simulink model "CONTROLLO_ADATTATIVO"  (R2020b)
settings: Solver=ode1  StartTime=0.0  StopTime=T(end)+3  FixedStep=0.001  RelTol=1e-3
undefined symbols (not defined in the file): a1, a2, d0, DiscIntNeverNeededParam, KD_ad, LAMBDA, param_esatti, pi0, q0
settings Model: Creator=pc  LastModifiedBy=Utente

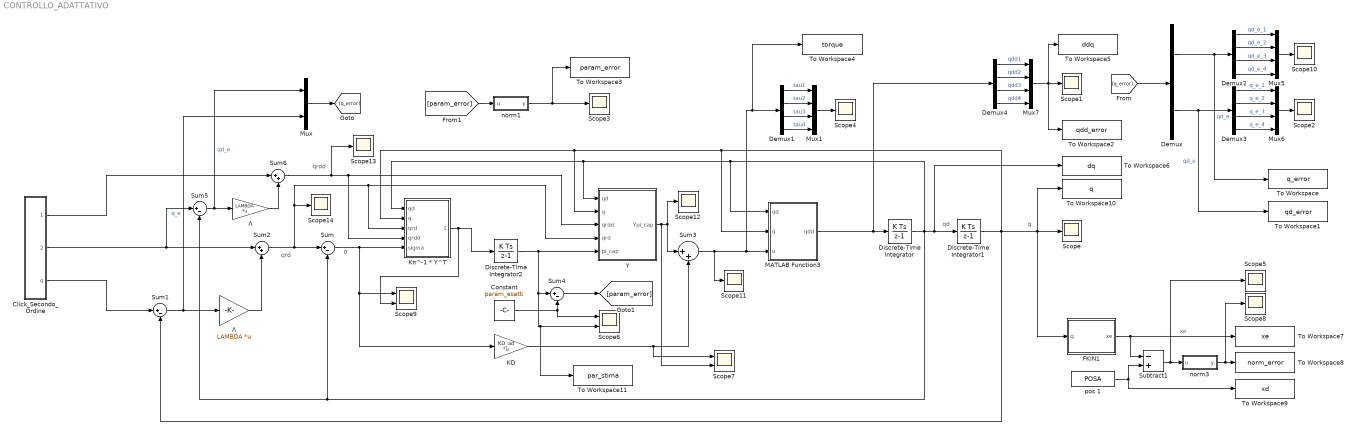
== system CONTROLLO_ADATTATIVO ==
  note: qd
  note: qrd
  note: qrdd
  note: q
  note: σ
  Click_Secondo_Ordine : Subsystem
  Constant : Constant  Value=param_esatti
  Demux : Demux  Outputs=2
  Demux{1..4} (4 alike) : Demux
  Discrete-Time Integrator : DiscreteIntegrator  InitialCondition=[0 0 0 0]  SampleTime=0.001  ICPrevOutput=DiscIntNeverNeededParam  ICPrevScaledInput=DiscIntNeverNeededParam
  Discrete-Time Integrator1 : DiscreteIntegrator  InitialCondition=q0  SampleTime=0.001  ICPrevOutput=DiscIntNeverNeededParam  ICPrevScaledInput=DiscIntNeverNeededParam
  Discrete-Time Integrator2 : DiscreteIntegrator  gainval=1  InitialCondition=pi0  SampleTime=0.001  ICPrevOutput=DiscIntNeverNeededParam  ICPrevScaledInput=DiscIntNeverNeededParam
  FKIN1 : MATLAB Function  TreatAsAtomicUnit=on
  KD : Gain  Gain=KD_ad  Multiplication=Matrix(K*u) (u vector)
  Kπ^-1 * Y^T : MATLAB Function  TreatAsAtomicUnit=on
  MATLAB Function3 : MATLAB Function  TreatAsAtomicUnit=on
  Mux : Mux  Inputs=2
  Mux{1,5..7} (4 alike) : Mux
  Scope{,1..5,8,10..14} (12 alike) : Scope
  Scope6 : Scope  NumInputPorts=2
  Scope7 : Scope  NumInputPorts=2
  Scope9 : Scope  NumInputPorts=2
  Subtract1 : Sum  Inputs=-+
  Sum{,1,4..5} (4 alike) : Sum  Inputs=|+-
  Sum2 : Sum  Inputs=|++
  Sum3 : Sum  Inputs=|++
  Sum6 : Sum  Inputs=|++
  To Workspace : ToWorkspace  VariableName=q_error  SaveFormat=Timeseries  SampleTime=-1
  To Workspace1 : ToWorkspace  VariableName=qd_error  SaveFormat=Timeseries  SampleTime=-1
  To Workspace10 : ToWorkspace  VariableName=q  SaveFormat=Timeseries  SampleTime=-1
  To Workspace11 : ToWorkspace  VariableName=par_stima  SaveFormat=Timeseries  SampleTime=-1
  To Workspace2 : ToWorkspace  VariableName=qdd_error  SaveFormat=Timeseries  SampleTime=-1
  To Workspace3 : ToWorkspace  VariableName=param_error  SaveFormat=Timeseries  SampleTime=-1
  To Workspace4 : ToWorkspace  VariableName=torque  SaveFormat=Timeseries  SampleTime=-1
  To Workspace5 : ToWorkspace  VariableName=ddq  SaveFormat=Timeseries  SampleTime=-1
  To Workspace6 : ToWorkspace  VariableName=dq  SaveFormat=Timeseries  SampleTime=-1
  To Workspace7 : ToWorkspace  VariableName=xe  SaveFormat=Timeseries  SampleTime=-1
  To Workspace8 : ToWorkspace  VariableName=norm_error  SaveFormat=Timeseries  SampleTime=-1
  To Workspace9 : ToWorkspace  VariableName=xd  SaveFormat=Timeseries  SampleTime=-1
  Y : MATLAB Function  TreatAsAtomicUnit=on
  norm1 : MATLAB Function  TreatAsAtomicUnit=on
  norm3 : MATLAB Function  TreatAsAtomicUnit=on
  pos 1 : FromWorkspace  VariableName=POSA  SampleTime=0.001  OutputAfterFinalValue=Holding final value
  Λ : Gain  Gain=LAMBDA  Multiplication=Matrix(K*u) (u vector)
  "Λ " : Gain  Gain=LAMBDA  Multiplication=Matrix(K*u) (u vector)
  wires:
  Sum6/1 -> Scope13/1, Y/3(qrdd), Kπ^-1 * Y^T/4(qrdd)
  Discrete-Time Integrator2/1 -> To Workspace11/1, Scope6/2, Sum4/1, Y/5(pi_cap)
  "Λ "/1 -> Sum6/2
  Kπ^-1 * Y^T/1(pi_capd) -> Scope9/2, Discrete-Time Integrator2/1
  Sum3/1 -> Scope11/1, To Workspace4/1, Demux1/1, MATLAB Function3/3(u)
  Y/1(Ypi_cap) -> Scope7/2, Sum3/1, Scope12/1
  Click_Secondo_Ordine/3(q) -> Sum1/1
  Sum/1 -> Scope9/1, KD/1, Kπ^-1 * Y^T/5(sigma)
  Click_Secondo_Ordine/2(q_d) -> Sum5/1, Sum2/1
  KD/1 -> Scope7/1, Sum3/2
  Λ/1 -> Sum2/2
  Click_Secondo_Ordine/1(q_dd) -> Sum6/1
  Sum2/1 -> Scope14/1, Y/4(qrd), Kπ^-1 * Y^T/3(qrd), Sum/1
  Demux4/1 -> Mux7/1  "qdd1"
  Demux4/2 -> Mux7/2  "qdd2"
  Demux4/3 -> Mux7/3  "qdd3"
  Demux1/3 -> Mux1/3  "tau3"
  Demux1/4 -> Mux1/4  "tau4"
  Mux1/1 -> Scope4/1
  Mux7/1 -> To Workspace5/1, To Workspace2/1, Scope1/1
  Discrete-Time Integrator/1 -> To Workspace6/1, Discrete-Time Integrator1/1, Y/1(qd), Kπ^-1 * Y^T/1(qd), MATLAB Function3/1(qd), Sum5/2, Sum/2
  Demux1/2 -> Mux1/2  "tau2"
  Demux4/4 -> Mux7/4  "qdd4"
  Demux1/1 -> Mux1/1  "tau1"
  MATLAB Function3/1(qdd) -> Demux4/1, Discrete-Time Integrator/1
  Mux/1 -> [q_error]
  Sum1/1 -> Mux/2, Λ/1  "q_e"
  Sum5/1 -> Mux/1, "Λ "/1  "qd_e"
  Mux6/1 -> Scope2/1
  Mux5/1 -> Scope10/1
  Demux3/3 -> Mux6/3  "q_e_3"
  Demux3/4 -> Mux6/4  "q_e_4"
  [q_error] -> Demux/1
  Demux3/1 -> Mux6/1  "q_e_1"
  Demux3/2 -> Mux6/2  "q_e_2"
  Demux2/3 -> Mux5/3  "qd_e_3"
  Demux2/4 -> Mux5/4  "qd_e_4"
  Demux/1 -> To Workspace/1, Demux2/1  "qd_e"
  Demux2/2 -> Mux5/2  "qd_e_2"
  Demux/2 -> To Workspace1/1, Demux3/1  "qd_e"
  Demux2/1 -> Mux5/1  "qd_e_1"
  Discrete-Time Integrator1/1 -> Y/2(q), Kπ^-1 * Y^T/2(q), MATLAB Function3/2(q), To Workspace10/1, FKIN1/1(q), Scope/1, Sum1/2
  [param_error] -> norm1/1(u)
  norm3/1(y) -> Scope8/1, To Workspace8/1
  pos 1/1 -> Subtract1/2, To Workspace9/1
  FKIN1/1(xe) -> Subtract1/1, To Workspace7/1  "xe"
  Subtract1/1 -> Scope5/1, norm3/1(u)
  Constant/1 -> Scope6/1, Sum4/2
  Sum4/1 -> [param_error]
  norm1/1(y) -> To Workspace3/1, Scope3/1

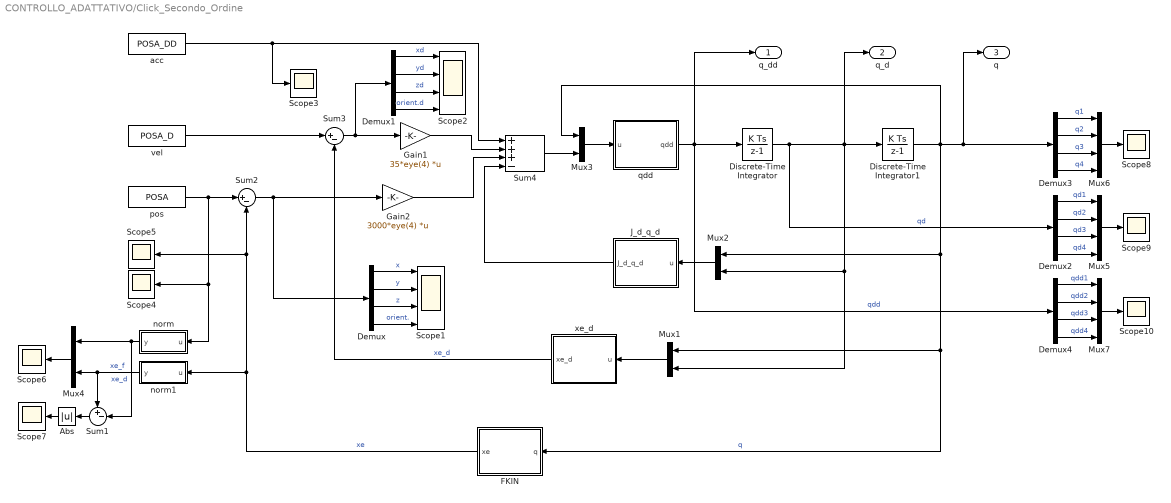
== system CONTROLLO_ADATTATIVO/Click_Secondo_Ordine ==
  Abs : Abs
  Demux{,1..4} (5 alike) : Demux
  Discrete-Time Integrator : DiscreteIntegrator  InitialCondition=zeros(1,4)  SampleTime=1e-3  ICPrevOutput=DiscIntNeverNeededParam  ICPrevScaledInput=DiscIntNeverNeededParam
  Discrete-Time Integrator1 : DiscreteIntegrator  InitialCondition=q0  SampleTime=1e-3  ICPrevOutput=DiscIntNeverNeededParam  ICPrevScaledInput=DiscIntNeverNeededParam
  FKIN : MATLAB Function  TreatAsAtomicUnit=on
  Gain1 : Gain  Gain=35*eye(4)  Multiplication=Matrix(K*u)
  Gain2 : Gain  Gain=3000*eye(4)  Multiplication=Matrix(K*u)
  J_d_q_d : MATLAB Function  TreatAsAtomicUnit=on
  Mux{1..4} (4 alike) : Mux  Inputs=2
  Mux5 : Mux
  Mux6 : Mux
  Mux7 : Mux
  Scope1 : Scope  NumInputPorts=4
  Scope{3..10} (8 alike) : Scope
  Scope2 : Scope  NumInputPorts=4
  Sum1 : Sum  Inputs=+-|
  Sum2 : Sum  Inputs=|+-
  Sum3 : Sum  Inputs=|+-
  Sum4 : Sum  Inputs=+++-
  acc : FromWorkspace  VariableName=POSA_DD  SampleTime=0.001
  norm : MATLAB Function  TreatAsAtomicUnit=on
  norm1 : MATLAB Function  TreatAsAtomicUnit=on
  "pos " : FromWorkspace  VariableName=POSA  SampleTime=0.001
  qdd : MATLAB Function  TreatAsAtomicUnit=on
  "vel " : FromWorkspace  VariableName=POSA_D  SampleTime=0.001
  xe_d : MATLAB Function  TreatAsAtomicUnit=on
  q_dd : Outport
  q_d : Outport  Port=2
  q : Outport  Port=3
  wires:
  Mux1/1 -> xe_d/1(u)
  J_d_q_d/1(J_d_q_d) -> Sum4/4
  "vel "/1 -> Sum3/1
  "pos "/1 -> norm/1(u), Scope4/1, Sum2/1
  Sum2/1 -> Demux/1, Gain2/1
  Sum3/1 -> Demux1/1, Gain1/1
  Discrete-Time Integrator1/1 -> Demux3/1, q/1, Mux3/1, Mux2/1, Mux1/1, FKIN/1(q)  "q"
  Mux2/1 -> J_d_q_d/1(u)
  xe_d/1(xe_d) -> Sum3/2  "xe_d"
  Mux3/1 -> qdd/1(u)
  Gain2/1 -> Sum4/3
  qdd/1(qdd) -> Demux4/1, q_dd/1, Discrete-Time Integrator/1  "qdd"
  FKIN/1(xe) -> Sum2/2, Scope5/1, norm1/1(u)  "xe"
  Discrete-Time Integrator/1 -> Demux2/1, q_d/1, Mux2/2, Mux1/2, Discrete-Time Integrator1/1  "qd"
  Sum4/1 -> Mux3/2
  acc/1 -> Sum4/1, Scope3/1
  Gain1/1 -> Sum4/2
  Abs/1 -> Scope7/1
  norm1/1(y) -> Sum1/1, Mux4/2  "xe_f"
  norm/1(y) -> Sum1/2, Mux4/1  "xe_d"
  Sum1/1 -> Abs/1
  Mux4/1 -> Scope6/1
  Demux/4 -> Scope1/4  "orient."
  Demux/2 -> Scope1/2  "y"
  Demux/1 -> Scope1/1  "x"
  Demux/3 -> Scope1/3  "z"
  Demux1/4 -> Scope2/4  "orient.d"
  Demux1/2 -> Scope2/2  "yd"
  Demux1/1 -> Scope2/1  "xd"
  Demux1/3 -> Scope2/3  "zd"
  Demux2/3 -> Mux5/3  "qd3"
  Demux3/1 -> Mux6/1  "q1"
  Mux5/1 -> Scope9/1
  Demux3/2 -> Mux6/2  "q2"
  Demux2/2 -> Mux5/2  "qd2"
  Demux3/4 -> Mux6/4  "q4"
  Demux2/1 -> Mux5/1  "qd1"
  Mux6/1 -> Scope8/1
  Demux3/3 -> Mux6/3  "q3"
  Demux2/4 -> Mux5/4  "qd4"
  Demux4/4 -> Mux7/4  "qdd4"
  Demux4/2 -> Mux7/2  "qdd2"
  Demux4/1 -> Mux7/1  "qdd1"
  Mux7/1 -> Scope10/1
  Demux4/3 -> Mux7/3  "qdd3"

== matlab function CONTROLLO_ADATTATIVO/Click_Secondo_Ordine/norm ==
  data: u input; y output
function y = norm(u)
y = norm(u);

== matlab function CONTROLLO_ADATTATIVO/Click_Secondo_Ordine/norm1 ==
  data: u input; y output
function y = norm(u)
y = norm(u);

== matlab function CONTROLLO_ADATTATIVO/norm3 ==
  data: u input; y output
function y = fcn(u)
y = norm(u);

== matlab function CONTROLLO_ADATTATIVO/Y ==
  data: qd input; q input; qrdd input; qrd input; pi_cap input; Ypi_cap output
function Ypi_cap = fcn(qd, q, qrdd, qrd, pi_cap)

q_1 = q(1);
q_2 = q(2);
q_3 = q(3);
q_4 = q(4);
qd_1 = qd(1);
qd_2 = qd(2);
qd_3 = qd(3);
qd_4 = qd(4);
q_rdd_1=qrdd(1);
q_rdd_2=qrdd(2);
q_rdd_3=qrdd(3);
q_rdd_4=qrdd(4);
q_rd_1=qrd(1);
q_rd_2=qrd(2);
q_rd_3=qrd(3);
q_rd_4=qrd(4);

Y=[q_rdd_1/16, q_rdd_1, q_rdd_1, q_rd_1, q_rdd_1*(cos(q_2)/4 + 5/16) + q_rdd_2*(cos(q_2)/8 + 1/16) - (q_rd_1*qd_2*sin(q_2))/8 - (q_rd_2*sin(q_2)*(qd_1 + qd_2))/8, q_rdd_1 + q_rdd_2, q_rdd_1 + q_rdd_2,      0, q_rdd_1*(cos(q_2)/2 + 1/2) + q_rdd_2*(cos(q_2)/4 + 1/4) - (q_rd_1*qd_2*sin(q_2))/4 - (q_rd_2*sin(q_2)*(qd_1 + qd_2))/4, q_rdd_1 + q_rdd_2,         q_rdd_1 + q_rdd_2 + 50*q_rdd_3,          0, q_rdd_1*(cos(q_2)/2 + 1/2) + q_rdd_2*(cos(q_2)/4 + 1/4) - (q_rd_1*qd_2*sin(q_2))/4 - (q_rd_2*sin(q_2)*(qd_1 + qd_2))/4, q_rdd_1 + q_rdd_2 + q_rdd_4,        q_rdd_1 + q_rdd_2 + 20*q_rdd_4,          0;
     0,       0,       0,      0,                                                      q_rdd_2/16 + q_rdd_1*(cos(q_2)/8 + 1/16) + (q_rd_1*qd_1*sin(q_2))/8, q_rdd_1 + q_rdd_2, q_rdd_1 + q_rdd_2, q_rd_2,                                                      q_rdd_2/4 + q_rdd_1*(cos(q_2)/4 + 1/4) + (q_rd_1*qd_1*sin(q_2))/4, q_rdd_1 + q_rdd_2,         q_rdd_1 + q_rdd_2 + 50*q_rdd_3,          0,                                                      q_rdd_2/4 + q_rdd_1*(cos(q_2)/4 + 1/4) + (q_rd_1*qd_1*sin(q_2))/4, q_rdd_1 + q_rdd_2 + q_rdd_4,        q_rdd_1 + q_rdd_2 + 20*q_rdd_4,          0;
     0,       0,       0,      0,                                                                                                                        0,                 0,                 0,      0,                                                                                                      q_rdd_3 + 981/100,                 0, 50*q_rdd_1 + 50*q_rdd_2 + 2500*q_rdd_3, 400*q_rd_3,                                                                                                      q_rdd_3 + 981/100,                           0,                                     0,          0;
        0,       0,       0,      0,                                                                                                                        0,                 0,                 0,      0,                                                                                                                      0,                 0,                                      0,          0,                                                                                                                      0, q_rdd_1 + q_rdd_2 + q_rdd_4, 20*q_rdd_1 + 20*q_rdd_2 + 400*q_rdd_4, 400*q_rd_4];

    
Ypi_cap = Y*pi_cap;

== matlab function CONTROLLO_ADATTATIVO/Kπ^-1 * Y^T ==
  data: qd input; q input; qrd input; qrdd input; sigma input; pi_capd output; Kpi parameter
function pi_capd = fcn(qd, q, qrd, qrdd, sigma, Kpi)

q_1 = q(1);
q_2 = q(2);
q_3 = q(3);
q_4 = q(4);
qd_1 = qd(1);
qd_2 = qd(2);
qd_3 = qd(3);
qd_4 = qd(4);
q_rd_1 = qrd(1);
q_rd_2 = qrd(2);
q_rd_3 = qrd(3);
q_rd_4 = qrd(4);
q_rdd_1 = qrdd(1);
q_rdd_2 = qrdd(2);
q_rdd_3 = qrdd(3);
q_rdd_4 = qrdd(4);

Y=[q_rdd_1/16, q_rdd_1, q_rdd_1, q_rd_1, q_rdd_1*(cos(q_2)/4 + 5/16) + q_rdd_2*(cos(q_2)/8 + 1/16) - (q_rd_1*qd_2*sin(q_2))/8 - (q_rd_2*sin(q_2)*(qd_1 + qd_2))/8, q_rdd_1 + q_rdd_2, q_rdd_1 + q_rdd_2,      0, q_rdd_1*(cos(q_2)/2 + 1/2) + q_rdd_2*(cos(q_2)/4 + 1/4) - (q_rd_1*qd_2*sin(q_2))/4 - (q_rd_2*sin(q_2)*(qd_1 + qd_2))/4, q_rdd_1 + q_rdd_2,         q_rdd_1 + q_rdd_2 + 50*q_rdd_3,          0, q_rdd_1*(cos(q_2)/2 + 1/2) + q_rdd_2*(cos(q_2)/4 + 1/4) - (q_rd_1*qd_2*sin(q_2))/4 - (q_rd_2*sin(q_2)*(qd_1 + qd_2))/4, q_rdd_1 + q_rdd_2 + q_rdd_4,        q_rdd_1 + q_rdd_2 + 20*q_rdd_4,          0;
     0,       0,       0,      0,                                                      q_rdd_2/16 + q_rdd_1*(cos(q_2)/8 + 1/16) + (q_rd_1*qd_1*sin(q_2))/8, q_rdd_1 + q_rdd_2, q_rdd_1 + q_rdd_2, q_rd_2,                                                      q_rdd_2/4 + q_rdd_1*(cos(q_2)/4 + 1/4) + (q_rd_1*qd_1*sin(q_2))/4, q_rdd_1 + q_rdd_2,         q_rdd_1 + q_rdd_2 + 50*q_rdd_3,          0,                                                      q_rdd_2/4 + q_rdd_1*(cos(q_2)/4 + 1/4) + (q_rd_1*qd_1*sin(q_2))/4, q_rdd_1 + q_rdd_2 + q_rdd_4,        q_rdd_1 + q_rdd_2 + 20*q_rdd_4,          0;
     0,       0,       0,      0,                                                                                                                        0,                 0,                 0,      0,                                                                                                      q_rdd_3 + 981/100,                 0, 50*q_rdd_1 + 50*q_rdd_2 + 2500*q_rdd_3, 400*q_rd_3,                                                                                                      q_rdd_3 + 981/100,                           0,                                     0,          0;
        0,       0,       0,      0,                                                                                                                        0,                 0,                 0,      0,                                                                                                                      0,                 0,                                      0,          0,                                                                                                                      0, q_rdd_1 + q_rdd_2 + q_rdd_4, 20*q_rdd_1 + 20*q_rdd_2 + 400*q_rdd_4, 400*q_rd_4];

    
pi_capd = inv(Kpi)* Y' * sigma;

== matlab function CONTROLLO_ADATTATIVO/FKIN1 ==
  data: q input; xe output; a2 parameter; a1 parameter; d0 parameter
function xe = fcn(q, a2, a1, d0)

theta1 = q(1);
theta2 = q(2);
d3 = q(3);
theta4 = q(4);

% Cinematica diretta
xe = [a1*cos(theta1)+a2*cos(theta1+theta2) ;
      a1*sin(theta1)+a2*sin(theta1+theta2) ;
      d3+d0;
      theta1+theta2+theta4; ];
end

== matlab function CONTROLLO_ADATTATIVO/MATLAB Function3 ==
  data: qd input; q input; u input; qdd output
function qdd = manipulator(qd, q, u)

q_1 = q(1);
q_2 = q(2);
q_3 = q(3);
q_4 = q(4);
qd_1 = qd(1);
qd_2 = qd(2);
qd_3 = qd(3);
qd_4 = qd(4);

l1 = 0.25;
l2 = 0.25;
ml1 = 25;   %Massa dal giunto 1 al giunto 2 .Non si considera quello della base.
ml2 = ml1;
ml3 = 10;
ml4 = 5; 


Il1 = 5;
Il2 = Il1;
Il3 = 0;
Il4 = 1;


mm = zeros(1,4);

%Costanti di trasmissione meccanica 
kr1 = 1;
kr2 = kr1;
kr3 = 50;
kr4 = 20;


Im1 = 0.02;
Im2 = Im1;
Im3 = 0.005;
Im4 = 0.001;


Fm1= 0.0001;
Fm2 = Fm1;
Fm3 = 0.01;
Fm4 = 0.005;

   
n = [ Fm1*qd_1 - (qd_2*sin(q_2)*(qd_1 + qd_2)*(ml2 + 2*ml3 + 2*ml4))/8 - qd_1*qd_2*sin(q_2)*(ml2/8 + ml3/4 + ml4/4);
                                                 sin(q_2)*(ml2/8 + ml3/4 + ml4/4)*qd_1^2 + Fm2*qd_2;
                                                                  (981*ml3)/100 + (981*ml4)/100 + 400*Fm3*qd_3;
                                                                             400*Fm4*qd_4];
 
                                                                    
B = [ Il1 + Il2 + Il3 + Il4 + Im1 + Im2 + Im3 + Im4 + ml1/16 + (5*ml2)/16 + ml3/2 + ml4/2 + (ml2*cos(q_2))/4 + (ml3*cos(q_2))/2 + (ml4*cos(q_2))/2, Il2 + Il3 + Il4 + Im2 + Im3 + Im4 + ml2/16 + ml3/4 + ml4/4 + (ml2*cos(q_2))/8 + (ml3*cos(q_2))/4 + (ml4*cos(q_2))/4,               50*Im3,  Il4 + 20*Im4;
                              Il2 + Il3 + Il4 + Im2 + Im3 + Im4 + ml2/16 + ml3/4 + ml4/4 + (ml2*cos(q_2))/8 + (ml3*cos(q_2))/4 + (ml4*cos(q_2))/4,                                                          Il2 + Il3 + Il4 + Im2 + Im3 + Im4 + ml2/16 + ml3/4 + ml4/4,               50*Im3,  Il4 + 20*Im4;
                                                                                           50*Im3,                                                                                                              50*Im3, 2500*Im3 + ml3 + ml4,             0;
                                                Il4 + 20*Im4,                                                                                                        Il4 + 20*Im4,                    0, Il4 + 400*Im4];
 
qdd = inv(B)*(u-n);

== matlab function CONTROLLO_ADATTATIVO/Click_Secondo_Ordine/FKIN ==
  data: q input; xe output; a2 parameter; a1 parameter; d0 parameter
function xe = fcn(q, a2, a1, d0)

theta1 = q(1);
theta2 = q(2);
d3 = q(3);
theta4 = q(4);

% Cinematica diretta
xe = [a1*cos(theta1)+a2*cos(theta1+theta2) ;
      a1*sin(theta1)+a2*sin(theta1+theta2) ;
      d3+d0;
      theta1+theta2+theta4];
end

== matlab function CONTROLLO_ADATTATIVO/Click_Secondo_Ordine/J_d_q_d ==
  data: u input; J_d_q_d output; a1 parameter; a2 parameter
function J_d_q_d = fcn(u, a1, a2)

q = u(1:4);
q1_d=u(5);
q2_d=u(6);
u2 = u(5:8);
% Jacobiano derivato

% J_d = [ -a1*cos(q(1))*q1_d+a2*cos(q(1)+q(2))*(q1_d+q2_d)   -a2*cos(q(1)+q(2))*(q1_d+q2_d)  0   0   ;
%        -a1*sin(q(1))*q1_d+a2*sin(q(1)+q(2))*(q1_d+q2_d)    -a2*sin(q(1)+q(2))*(q1_d+q2_d)  0   0   ;
%                    0                              0        0    0   ;
%                    0                              0         0   0   ];
               
               
J_d = [ (-q1_d + q2_d)*(a2*cos(q(1)+q(2)))-q1_d*a1*cos(q(1)),  -(q1_d+q2_d)*(a2*cos(q(1)+q(2))),   0,  0;
         -(q1_d+q2_d)*(a2*sin(q(1)+q(2)))-q1_d*a1*sin(q(1)),   -(q1_d+q2_d)*(a2*sin(q(1)+q(2))),   0,  0;
         0, 0, 0, 0;
         0, 0, 0, 0;];
     
               
    J_d_q_d = J_d*u2;
end

== matlab function CONTROLLO_ADATTATIVO/Click_Secondo_Ordine/qdd ==
  data: u input; qdd output; a1 parameter; a2 parameter
function qdd = fcn(u, a1, a2)

q = u(1:4);
u2 = u(5:8);

% Jacobiano
J = [ -a1*sin(q(1))-a2*sin(q(1)+q(2))   -a2*sin(q(1)+q(2))  0   0   ;
       a1*cos(q(1))+a2*cos(q(1)+q(2))    a2*cos(q(1)+q(2))  0   0   ;
                   0                              0         1   0   ;
                   1                              1         0   1   ];

qdd = inv(J)*(u2);
end

== matlab function CONTROLLO_ADATTATIVO/Click_Secondo_Ordine/xe_d ==
  data: u input; xe_d output; a1 parameter; a2 parameter
function xe_d = fcn(u, a1, a2)

q = u(1:4);
u2 = u(5:8);

% Jacobiano
J = [ -a1*sin(q(1))-a2*sin(q(1)+q(2))   -a2*sin(q(1)+q(2))  0   0   ;
       a1*cos(q(1))+a2*cos(q(1)+q(2))    a2*cos(q(1)+q(2))  0   0   ;
                   0                              0         1   0   ;
                   1                              1         0   1   ];
               
    xe_d = J*u2;
end

== matlab function CONTROLLO_ADATTATIVO/norm1 ==
  data: u input; y output
function y = fcn(u)
y = norm(u);
